simulink library "TYPEBP_MASTER_tmp"  (Simulink 8.6)
settings: Solver=ode45  StartTime=0.0  StopTime=10.0  RelTol=1e-3
undefined symbols (not defined in the file): TYPEC, TYPEC_MASTER
libraries: cdsEpicsOut x112, cdsFilt x79, cdsTP x59, cdsFiltCtrl x36, VIS_LIB x20, cdsEpicsIn x18, cdsMuxMatrix x14, STATE_BIO_MASTER x12, cdsEpicsBinIn x8, cdsFunctionCall x4, lockin x4, cdsEpicsStringIn x2
(part 5 of 13)

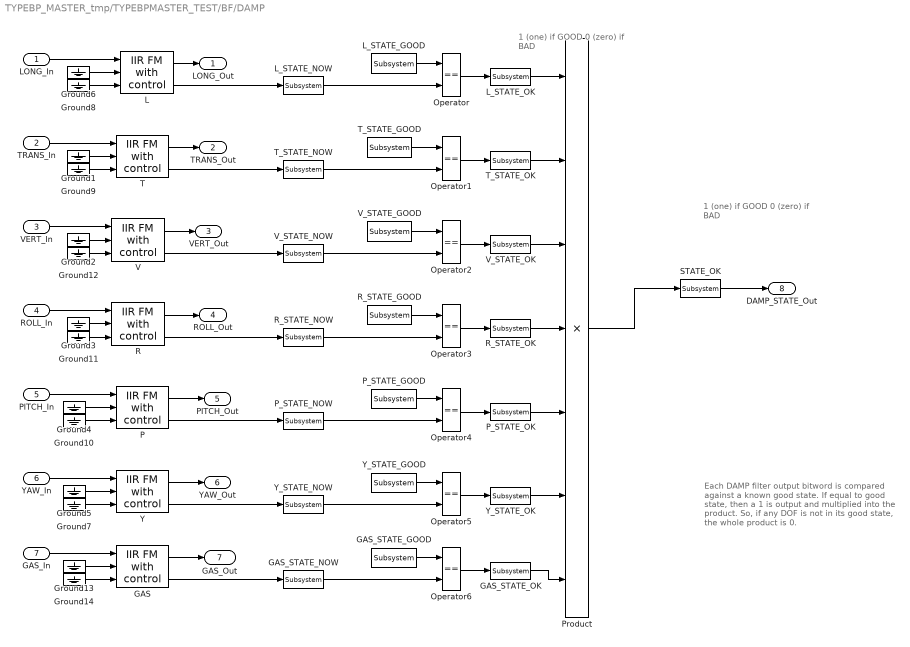
== system TYPEBP_MASTER_tmp/TYPEBPMASTER_TEST/BF/DAMP ==
  note: Each DAMP filter output bitword is
      | compared against a known good state.
      | If equal to good state, then a 1 is output
      | and multiplied into the product. So, if any DOF
      | is not in its good state, the whole product is 0.
  note: 1 (one) if GOOD
      | 0 (zero) if BAD
  note: 1 (one) if GOOD
      | 0 (zero) if BAD
  LONG_In : Inport
  TRANS_In : Inport  Port=2
  VERT_In : Inport  Port=3
  ROLL_In : Inport  Port=4
  PITCH_In : Inport  Port=5
  YAW_In : Inport  Port=6
  GAS_In : Inport  Port=7
  GAS : cdsFiltCtrl/IIR FM with control  Tag=cdsFiltCtrl  Description=|
      | cdsFiltCntrl is the standard IIR filter module (exactly the same as cdsFilt) but with added control data output 'Ctrl'. Filter module digital signal output appears on the first output, which is called 'Val'. 'Ctrl' output has a bit pattern encoding the state of filter's on/off switches (FM1 through FM10). The bit values are:
      |                                                                                                                                                                                                                                                                                                                                       
      | module 	hex	dec                                                                                                                                                                                                                                                                                                                       
      | -----------------------                                                                                                                                                                                                                                                                                                               
      | FM1	0x20                    32                                                                                                                                                                                                                                                                                                        
      | FM2	0x80                     128                                                                                                                                                                                                                                                                                                      
      | FM3	0x200                   512                                                                                                                                                                                                                                                                                                       
      | FM4	0x800                   2048                                                                                                                                                                                                                                                                                                      
      | FM5	0x2000                 8192                                                                                                                                                                                                                                                                                                       
      | FM6	0x8000                 32768                                                                                                                                                                                                                                                                                                      
      | FM7	0x20000                131072                                                                                                                                                                                                                                                                                                     
      | FM8	0x80000                 524288                                                                                                                                                                                                                                                                                                    
      | FM9	0x200000               2097152                                                                                                                                                                                                                                                                                                    
      | FM10	0x800000               8388608                                                                                                                                                                                                                                                                                                   
      |                                                                                                                                                                                                                                                                                                                                       
      | This bit data can be used to drive some other switches or it can be output using a binary I/O module.
      settings: AttributesFormatString=%<Tag>
  GAS_STATE_GOOD : cdsEpicsIn/Subsystem  Tag=cdsEpicsIn  Description=|
      | Purpose:                                                                              
      | Create an EPICS input channel connection to the FE realtime controls.                 
      |                                                                                       
      | Operation:                                                                            
      | Outputs value from an EPICS ai record. Value is floating point with a precision of 3..
      |                                                                                       
      | Usage:                                                                                
      | Name the part with the desired EPICS channel name.
      settings: AttributesFormatString=%<Tag>
  GAS_STATE_NOW : cdsEpicsOut/Subsystem  Tag=cdsEpicsOutput  Description=|
      | Purpose:                                          
      | Output a FE signal to an EPICS channel.           
      |                                                   
      | Operation:                                        
      | Takes input value and passes it to EPICS record.  
      |                                                   
      | Usage:                                            
      | Name the part with the desired EPICS rrecord name.
      settings: AttributesFormatString=%<Tag>
  GAS_STATE_OK : cdsEpicsOut/Subsystem  Tag=cdsEpicsOutput  Description=|
      | Purpose:                                          
      | Output a FE signal to an EPICS channel.           
      |                                                   
      | Operation:                                        
      | Takes input value and passes it to EPICS record.  
      |                                                   
      | Usage:                                            
      | Name the part with the desired EPICS rrecord name.
      settings: AttributesFormatString=%<Tag>
  Ground{1..14} (14 alike) : Ground
  L : cdsFiltCtrl/IIR FM with control  Tag=cdsFiltCtrl  Description=|
      | cdsFiltCntrl is the standard IIR filter module (exactly the same as cdsFilt) but with added control data output 'Ctrl'. Filter module digital signal output appears on the first output, which is called 'Val'. 'Ctrl' output has a bit pattern encoding the state of filter's on/off switches (FM1 through FM10). The bit values are:
      |                                                                                                                                                                                                                                                                                                                                       
      | module 	hex	dec                                                                                                                                                                                                                                                                                                                       
      | -----------------------                                                                                                                                                                                                                                                                                                               
      | FM1	0x20                    32                                                                                                                                                                                                                                                                                                        
      | FM2	0x80                     128                                                                                                                                                                                                                                                                                                      
      | FM3	0x200                   512                                                                                                                                                                                                                                                                                                       
      | FM4	0x800                   2048                                                                                                                                                                                                                                                                                                      
      | FM5	0x2000                 8192                                                                                                                                                                                                                                                                                                       
      | FM6	0x8000                 32768                                                                                                                                                                                                                                                                                                      
      | FM7	0x20000                131072                                                                                                                                                                                                                                                                                                     
      | FM8	0x80000                 524288                                                                                                                                                                                                                                                                                                    
      | FM9	0x200000               2097152                                                                                                                                                                                                                                                                                                    
      | FM10	0x800000               8388608                                                                                                                                                                                                                                                                                                   
      |                                                                                                                                                                                                                                                                                                                                       
      | This bit data can be used to drive some other switches or it can be output using a binary I/O module.
      settings: AttributesFormatString=%<Tag>
  L_STATE_GOOD : cdsEpicsIn/Subsystem  Tag=cdsEpicsIn  Description=|
      | Purpose:                                                                              
      | Create an EPICS input channel connection to the FE realtime controls.                 
      |                                                                                       
      | Operation:                                                                            
      | Outputs value from an EPICS ai record. Value is floating point with a precision of 3..
      |                                                                                       
      | Usage:                                                                                
      | Name the part with the desired EPICS channel name.
      settings: AttributesFormatString=%<Tag>
  L_STATE_NOW : cdsEpicsOut/Subsystem  Tag=cdsEpicsOutput  Description=|
      | Purpose:                                          
      | Output a FE signal to an EPICS channel.           
      |                                                   
      | Operation:                                        
      | Takes input value and passes it to EPICS record.  
      |                                                   
      | Usage:                                            
      | Name the part with the desired EPICS rrecord name.
      settings: AttributesFormatString=%<Tag>
  L_STATE_OK : cdsEpicsOut/Subsystem  Tag=cdsEpicsOutput  Description=|
      | Purpose:                                          
      | Output a FE signal to an EPICS channel.           
      |                                                   
      | Operation:                                        
      | Takes input value and passes it to EPICS record.  
      |                                                   
      | Usage:                                            
      | Name the part with the desired EPICS rrecord name.
      settings: AttributesFormatString=%<Tag>
  Operator{,1..6} (7 alike) : RelationalOperator  Operator===  OutDataTypeStr=boolean
  P : cdsFiltCtrl/IIR FM with control  Tag=cdsFiltCtrl  Description=|
      | cdsFiltCntrl is the standard IIR filter module (exactly the same as cdsFilt) but with added control data output 'Ctrl'. Filter module digital signal output appears on the first output, which is called 'Val'. 'Ctrl' output has a bit pattern encoding the state of filter's on/off switches (FM1 through FM10). The bit values are:
      |                                                                                                                                                                                                                                                                                                                                       
      | module 	hex	dec                                                                                                                                                                                                                                                                                                                       
      | -----------------------                                                                                                                                                                                                                                                                                                               
      | FM1	0x20                    32                                                                                                                                                                                                                                                                                                        
      | FM2	0x80                     128                                                                                                                                                                                                                                                                                                      
      | FM3	0x200                   512                                                                                                                                                                                                                                                                                                       
      | FM4	0x800                   2048                                                                                                                                                                                                                                                                                                      
      | FM5	0x2000                 8192                                                                                                                                                                                                                                                                                                       
      | FM6	0x8000                 32768                                                                                                                                                                                                                                                                                                      
      | FM7	0x20000                131072                                                                                                                                                                                                                                                                                                     
      | FM8	0x80000                 524288                                                                                                                                                                                                                                                                                                    
      | FM9	0x200000               2097152                                                                                                                                                                                                                                                                                                    
      | FM10	0x800000               8388608                                                                                                                                                                                                                                                                                                   
      |                                                                                                                                                                                                                                                                                                                                       
      | This bit data can be used to drive some other switches or it can be output using a binary I/O module.
      settings: AttributesFormatString=%<Tag>
  P_STATE_GOOD : cdsEpicsIn/Subsystem  Tag=cdsEpicsIn  Description=|
      | Purpose:                                                                              
      | Create an EPICS input channel connection to the FE realtime controls.                 
      |                                                                                       
      | Operation:                                                                            
      | Outputs value from an EPICS ai record. Value is floating point with a precision of 3..
      |                                                                                       
      | Usage:                                                                                
      | Name the part with the desired EPICS channel name.
      settings: AttributesFormatString=%<Tag>
  P_STATE_NOW : cdsEpicsOut/Subsystem  Tag=cdsEpicsOutput  Description=|
      | Purpose:                                          
      | Output a FE signal to an EPICS channel.           
      |                                                   
      | Operation:                                        
      | Takes input value and passes it to EPICS record.  
      |                                                   
      | Usage:                                            
      | Name the part with the desired EPICS rrecord name.
      settings: AttributesFormatString=%<Tag>
  P_STATE_OK : cdsEpicsOut/Subsystem  Tag=cdsEpicsOutput  Description=|
      | Purpose:                                          
      | Output a FE signal to an EPICS channel.           
      |                                                   
      | Operation:                                        
      | Takes input value and passes it to EPICS record.  
      |                                                   
      | Usage:                                            
      | Name the part with the desired EPICS rrecord name.
      settings: AttributesFormatString=%<Tag>
  Product : Product  Inputs=7  RndMeth=Zero
  R : cdsFiltCtrl/IIR FM with control  Tag=cdsFiltCtrl  Description=|
      | cdsFiltCntrl is the standard IIR filter module (exactly the same as cdsFilt) but with added control data output 'Ctrl'. Filter module digital signal output appears on the first output, which is called 'Val'. 'Ctrl' output has a bit pattern encoding the state of filter's on/off switches (FM1 through FM10). The bit values are:
      |                                                                                                                                                                                                                                                                                                                                       
      | module 	hex	dec                                                                                                                                                                                                                                                                                                                       
      | -----------------------                                                                                                                                                                                                                                                                                                               
      | FM1	0x20                    32                                                                                                                                                                                                                                                                                                        
      | FM2	0x80                     128                                                                                                                                                                                                                                                                                                      
      | FM3	0x200                   512                                                                                                                                                                                                                                                                                                       
      | FM4	0x800                   2048                                                                                                                                                                                                                                                                                                      
      | FM5	0x2000                 8192                                                                                                                                                                                                                                                                                                       
      | FM6	0x8000                 32768                                                                                                                                                                                                                                                                                                      
      | FM7	0x20000                131072                                                                                                                                                                                                                                                                                                     
      | FM8	0x80000                 524288                                                                                                                                                                                                                                                                                                    
      | FM9	0x200000               2097152                                                                                                                                                                                                                                                                                                    
      | FM10	0x800000               8388608                                                                                                                                                                                                                                                                                                   
      |                                                                                                                                                                                                                                                                                                                                       
      | This bit data can be used to drive some other switches or it can be output using a binary I/O module.
      settings: AttributesFormatString=%<Tag>
  R_STATE_GOOD : cdsEpicsIn/Subsystem  Tag=cdsEpicsIn  Description=|
      | Purpose:                                                                              
      | Create an EPICS input channel connection to the FE realtime controls.                 
      |                                                                                       
      | Operation:                                                                            
      | Outputs value from an EPICS ai record. Value is floating point with a precision of 3..
      |                                                                                       
      | Usage:                                                                                
      | Name the part with the desired EPICS channel name.
      settings: AttributesFormatString=%<Tag>
  R_STATE_NOW : cdsEpicsOut/Subsystem  Tag=cdsEpicsOutput  Description=|
      | Purpose:                                          
      | Output a FE signal to an EPICS channel.           
      |                                                   
      | Operation:                                        
      | Takes input value and passes it to EPICS record.  
      |                                                   
      | Usage:                                            
      | Name the part with the desired EPICS rrecord name.
      settings: AttributesFormatString=%<Tag>
  R_STATE_OK : cdsEpicsOut/Subsystem  Tag=cdsEpicsOutput  Description=|
      | Purpose:                                          
      | Output a FE signal to an EPICS channel.           
      |                                                   
      | Operation:                                        
      | Takes input value and passes it to EPICS record.  
      |                                                   
      | Usage:                                            
      | Name the part with the desired EPICS rrecord name.
      settings: AttributesFormatString=%<Tag>
  STATE_OK : cdsEpicsOut/Subsystem  Tag=cdsEpicsOutput  Description=|
      | Purpose:                                          
      | Output a FE signal to an EPICS channel.           
      |                                                   
      | Operation:                                        
      | Takes input value and passes it to EPICS record.  
      |                                                   
      | Usage:                                            
      | Name the part with the desired EPICS rrecord name.
      settings: AttributesFormatString=%<Tag>
  T : cdsFiltCtrl/IIR FM with control  Tag=cdsFiltCtrl  Description=|
      | cdsFiltCntrl is the standard IIR filter module (exactly the same as cdsFilt) but with added control data output 'Ctrl'. Filter module digital signal output appears on the first output, which is called 'Val'. 'Ctrl' output has a bit pattern encoding the state of filter's on/off switches (FM1 through FM10). The bit values are:
      |                                                                                                                                                                                                                                                                                                                                       
      | module 	hex	dec                                                                                                                                                                                                                                                                                                                       
      | -----------------------                                                                                                                                                                                                                                                                                                               
      | FM1	0x20                    32                                                                                                                                                                                                                                                                                                        
      | FM2	0x80                     128                                                                                                                                                                                                                                                                                                      
      | FM3	0x200                   512                                                                                                                                                                                                                                                                                                       
      | FM4	0x800                   2048                                                                                                                                                                                                                                                                                                      
      | FM5	0x2000                 8192                                                                                                                                                                                                                                                                                                       
      | FM6	0x8000                 32768                                                                                                                                                                                                                                                                                                      
      | FM7	0x20000                131072                                                                                                                                                                                                                                                                                                     
      | FM8	0x80000                 524288                                                                                                                                                                                                                                                                                                    
      | FM9	0x200000               2097152                                                                                                                                                                                                                                                                                                    
      | FM10	0x800000               8388608                                                                                                                                                                                                                                                                                                   
      |                                                                                                                                                                                                                                                                                                                                       
      | This bit data can be used to drive some other switches or it can be output using a binary I/O module.
      settings: AttributesFormatString=%<Tag>
  T_STATE_GOOD : cdsEpicsIn/Subsystem  Tag=cdsEpicsIn  Description=|
      | Purpose:                                                                              
      | Create an EPICS input channel connection to the FE realtime controls.                 
      |                                                                                       
      | Operation:                                                                            
      | Outputs value from an EPICS ai record. Value is floating point with a precision of 3..
      |                                                                                       
      | Usage:                                                                                
      | Name the part with the desired EPICS channel name.
      settings: AttributesFormatString=%<Tag>
  T_STATE_NOW : cdsEpicsOut/Subsystem  Tag=cdsEpicsOutput  Description=|
      | Purpose:                                          
      | Output a FE signal to an EPICS channel.           
      |                                                   
      | Operation:                                        
      | Takes input value and passes it to EPICS record.  
      |                                                   
      | Usage:                                            
      | Name the part with the desired EPICS rrecord name.
      settings: AttributesFormatString=%<Tag>
  T_STATE_OK : cdsEpicsOut/Subsystem  Tag=cdsEpicsOutput  Description=|
      | Purpose:                                          
      | Output a FE signal to an EPICS channel.           
      |                                                   
      | Operation:                                        
      | Takes input value and passes it to EPICS record.  
      |                                                   
      | Usage:                                            
      | Name the part with the desired EPICS rrecord name.
      settings: AttributesFormatString=%<Tag>
  V : cdsFiltCtrl/IIR FM with control  Tag=cdsFiltCtrl  Description=|
      | cdsFiltCntrl is the standard IIR filter module (exactly the same as cdsFilt) but with added control data output 'Ctrl'. Filter module digital signal output appears on the first output, which is called 'Val'. 'Ctrl' output has a bit pattern encoding the state of filter's on/off switches (FM1 through FM10). The bit values are:
      |                                                                                                                                                                                                                                                                                                                                       
      | module 	hex	dec                                                                                                                                                                                                                                                                                                                       
      | -----------------------                                                                                                                                                                                                                                                                                                               
      | FM1	0x20                    32                                                                                                                                                                                                                                                                                                        
      | FM2	0x80                     128                                                                                                                                                                                                                                                                                                      
      | FM3	0x200                   512                                                                                                                                                                                                                                                                                                       
      | FM4	0x800                   2048                                                                                                                                                                                                                                                                                                      
      | FM5	0x2000                 8192                                                                                                                                                                                                                                                                                                       
      | FM6	0x8000                 32768                                                                                                                                                                                                                                                                                                      
      | FM7	0x20000                131072                                                                                                                                                                                                                                                                                                     
      | FM8	0x80000                 524288                                                                                                                                                                                                                                                                                                    
      | FM9	0x200000               2097152                                                                                                                                                                                                                                                                                                    
      | FM10	0x800000               8388608                                                                                                                                                                                                                                                                                                   
      |                                                                                                                                                                                                                                                                                                                                       
      | This bit data can be used to drive some other switches or it can be output using a binary I/O module.
      settings: AttributesFormatString=%<Tag>
  V_STATE_GOOD : cdsEpicsIn/Subsystem  Tag=cdsEpicsIn  Description=|
      | Purpose:                                                                              
      | Create an EPICS input channel connection to the FE realtime controls.                 
      |                                                                                       
      | Operation:                                                                            
      | Outputs value from an EPICS ai record. Value is floating point with a precision of 3..
      |                                                                                       
      | Usage:                                                                                
      | Name the part with the desired EPICS channel name.
      settings: AttributesFormatString=%<Tag>
  V_STATE_NOW : cdsEpicsOut/Subsystem  Tag=cdsEpicsOutput  Description=|
      | Purpose:                                          
      | Output a FE signal to an EPICS channel.           
      |                                                   
      | Operation:                                        
      | Takes input value and passes it to EPICS record.  
      |                                                   
      | Usage:                                            
      | Name the part with the desired EPICS rrecord name.
      settings: AttributesFormatString=%<Tag>
  V_STATE_OK : cdsEpicsOut/Subsystem  Tag=cdsEpicsOutput  Description=|
      | Purpose:                                          
      | Output a FE signal to an EPICS channel.           
      |                                                   
      | Operation:                                        
      | Takes input value and passes it to EPICS record.  
      |                                                   
      | Usage:                                            
      | Name the part with the desired EPICS rrecord name.
      settings: AttributesFormatString=%<Tag>
  Y : cdsFiltCtrl/IIR FM with control  Tag=cdsFiltCtrl  Description=|
      | cdsFiltCntrl is the standard IIR filter module (exactly the same as cdsFilt) but with added control data output 'Ctrl'. Filter module digital signal output appears on the first output, which is called 'Val'. 'Ctrl' output has a bit pattern encoding the state of filter's on/off switches (FM1 through FM10). The bit values are:
      |                                                                                                                                                                                                                                                                                                                                       
      | module 	hex	dec                                                                                                                                                                                                                                                                                                                       
      | -----------------------                                                                                                                                                                                                                                                                                                               
      | FM1	0x20                    32                                                                                                                                                                                                                                                                                                        
      | FM2	0x80                     128                                                                                                                                                                                                                                                                                                      
      | FM3	0x200                   512                                                                                                                                                                                                                                                                                                       
      | FM4	0x800                   2048                                                                                                                                                                                                                                                                                                      
      | FM5	0x2000                 8192                                                                                                                                                                                                                                                                                                       
      | FM6	0x8000                 32768                                                                                                                                                                                                                                                                                                      
      | FM7	0x20000                131072                                                                                                                                                                                                                                                                                                     
      | FM8	0x80000                 524288                                                                                                                                                                                                                                                                                                    
      | FM9	0x200000               2097152                                                                                                                                                                                                                                                                                                    
      | FM10	0x800000               8388608                                                                                                                                                                                                                                                                                                   
      |                                                                                                                                                                                                                                                                                                                                       
      | This bit data can be used to drive some other switches or it can be output using a binary I/O module.
      settings: AttributesFormatString=%<Tag>
  Y_STATE_GOOD : cdsEpicsIn/Subsystem  Tag=cdsEpicsIn  Description=|
      | Purpose:                                                                              
      | Create an EPICS input channel connection to the FE realtime controls.                 
      |                                                                                       
      | Operation:                                                                            
      | Outputs value from an EPICS ai record. Value is floating point with a precision of 3..
      |                                                                                       
      | Usage:                                                                                
      | Name the part with the desired EPICS channel name.
      settings: AttributesFormatString=%<Tag>
  Y_STATE_NOW : cdsEpicsOut/Subsystem  Tag=cdsEpicsOutput  Description=|
      | Purpose:                                          
      | Output a FE signal to an EPICS channel.           
      |                                                   
      | Operation:                                        
      | Takes input value and passes it to EPICS record.  
      |                                                   
      | Usage:                                            
      | Name the part with the desired EPICS rrecord name.
      settings: AttributesFormatString=%<Tag>
  Y_STATE_OK : cdsEpicsOut/Subsystem  Tag=cdsEpicsOutput  Description=|
      | Purpose:                                          
      | Output a FE signal to an EPICS channel.           
      |                                                   
      | Operation:                                        
      | Takes input value and passes it to EPICS record.  
      |                                                   
      | Usage:                                            
      | Name the part with the desired EPICS rrecord name.
      settings: AttributesFormatString=%<Tag>
  LONG_Out : Outport
  TRANS_Out : Outport  Port=2
  VERT_Out : Outport  Port=3
  ROLL_Out : Outport  Port=4
  PITCH_Out : Outport  Port=5
  YAW_Out : Outport  Port=6
  GAS_Out : Outport  Port=7
  DAMP_STATE_Out : Outport  Port=8
  wires:
  GAS/1 -> GAS_Out/1
  STATE_OK/1 -> DAMP_STATE_Out/1
  Ground13/1 -> GAS/2
  GAS_In/1 -> GAS/1
  GAS_STATE_GOOD/1 -> Operator6/1
  GAS/2 -> GAS_STATE_NOW/1
  Operator6/1 -> GAS_STATE_OK/1
  GAS_STATE_OK/1 -> Product/7
  GAS_STATE_NOW/1 -> Operator6/2
  Ground14/1 -> GAS/3
  R/1 -> ROLL_Out/1
  P/1 -> PITCH_Out/1
  Y/1 -> YAW_Out/1
  Ground6/1 -> L/2
  Ground1/1 -> T/2
  Ground2/1 -> V/2
  Ground3/1 -> R/2
  Ground4/1 -> P/2
  Ground5/1 -> Y/2
  LONG_In/1 -> L/1
  L/1 -> LONG_Out/1
  YAW_In/1 -> Y/1
  V/1 -> VERT_Out/1
  T/1 -> TRANS_Out/1
  PITCH_In/1 -> P/1
  ROLL_In/1 -> R/1
  VERT_In/1 -> V/1
  TRANS_In/1 -> T/1
  L_STATE_GOOD/1 -> Operator/1
  L/2 -> L_STATE_NOW/1
  T_STATE_GOOD/1 -> Operator1/1
  T/2 -> T_STATE_NOW/1
  V_STATE_GOOD/1 -> Operator2/1
  V/2 -> V_STATE_NOW/1
  R_STATE_GOOD/1 -> Operator3/1
  R/2 -> R_STATE_NOW/1
  P_STATE_GOOD/1 -> Operator4/1
  P/2 -> P_STATE_NOW/1
  Y_STATE_GOOD/1 -> Operator5/1
  Y/2 -> Y_STATE_NOW/1
  Product/1 -> STATE_OK/1
  Operator/1 -> L_STATE_OK/1
  Operator1/1 -> T_STATE_OK/1
  Operator2/1 -> V_STATE_OK/1
  Operator3/1 -> R_STATE_OK/1
  Operator4/1 -> P_STATE_OK/1
  Operator5/1 -> Y_STATE_OK/1
  L_STATE_OK/1 -> Product/1
  T_STATE_OK/1 -> Product/2
  V_STATE_OK/1 -> Product/3
  R_STATE_OK/1 -> Product/4
  P_STATE_OK/1 -> Product/5
  Y_STATE_OK/1 -> Product/6
  L_STATE_NOW/1 -> Operator/2
  T_STATE_NOW/1 -> Operator1/2
  V_STATE_NOW/1 -> Operator2/2
  R_STATE_NOW/1 -> Operator3/2
  P_STATE_NOW/1 -> Operator4/2
  Y_STATE_NOW/1 -> Operator5/2
  Ground7/1 -> Y/3
  Ground8/1 -> L/3
  Ground9/1 -> T/3
  Ground10/1 -> P/3
  Ground11/1 -> R/3
  Ground12/1 -> V/3
